simulink model "td"  (R2022b)
settings: Solver=ode4  StartTime=0.0  StopTime=10.0  FixedStep=0.01  RelTol=1e-3
settings Model: Creator=Administrator  LastModifiedBy=Administrator

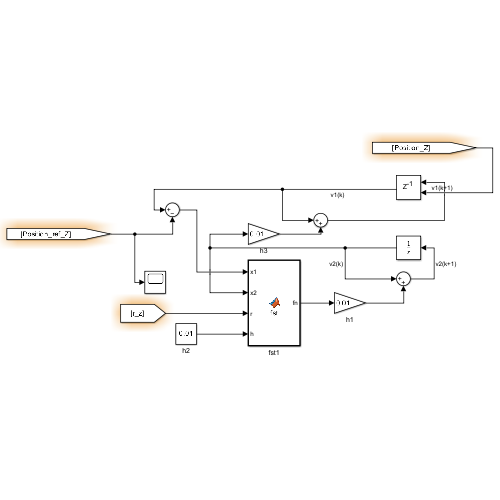
[thumbnail: Simulink's stored preview of the top-level diagram]
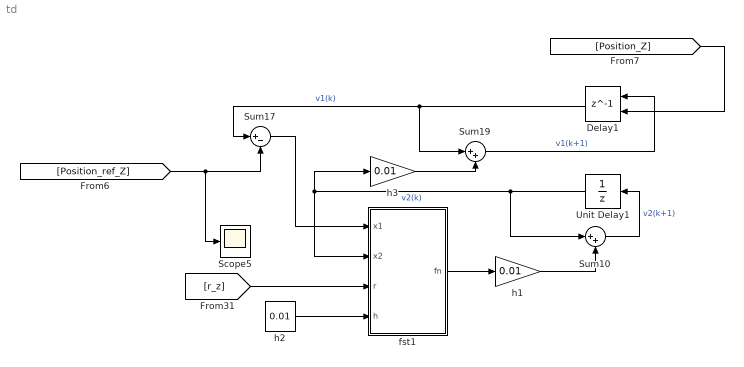
== system td ==
  Delay1 : Delay  DelayLength=1  InitialConditionSource=Input port
      settings: InputPortMap=u0,p4
  Scope5 : Scope
  Sum10 : Sum  Inputs=|++
  Sum17 : Sum  Inputs=|+-
  Sum19 : Sum  Inputs=|++
  Unit Delay1 : UnitDelay  SampleTime=-1  HasFrameUpgradeWarning=on
  fst1 : MATLAB Function  TreatAsAtomicUnit=on
  h1 : Gain  Gain=0.01
  h2 : Constant  Value=0.01
  h3 : Gain  Gain=0.01
  wires:
  Sum10/1 -> Unit Delay1/1  "v2(k+1)"
  [Position_Z] -> Delay1/2
  h3/1 -> Sum19/2
  fst1/1(fn) -> h1/1
  Sum17/1 -> fst1/1(x1)
  [r_z] -> fst1/3(r)
  h1/1 -> Sum10/2
  Sum19/1 -> Delay1/1  "v1(k+1)"
  [Position_ref_Z] -> Scope5/1, Sum17/2
  Delay1/1 -> Sum19/1, Sum17/1  "v1(k)"
  h2/1 -> fst1/4(h)
  Unit Delay1/1 -> Sum10/1, fst1/2(x2), h3/1  "v2(k)"

== matlab function td/fst1 ==
  data: x1 input; fn output; x2 input; r input; h input
%fst函数
function fn=fst(x1,x2,r,h)
d=h*r;
d0=h*d;
y=x1+h*x2;
a0=sqrt(d^2+8*r*abs(y));
if abs(y)<=d0
    a=x2+y/h;
else
    a=x2+0.5*(a0-d)*sgn(y);
end
fn=-r*sat(a,d);
end
%符号函数
function y=sgn(x)
if x>0
    y=1;
elseif x<0
    y=-1;
else
    y=0;
end
end
%sat函数
function y=sat(a,d)
if abs(a)<=d
    y=a/d;
else
    y=sgn(a);
end
end
%符号函数
